simulink model "Pendulum_Model"  (R2015a)
settings: Solver=ode45  StartTime=0.0  StopTime=50  RelTol=1e-3
undefined symbols (not defined in the file or in its folder): F_fan, g, k, l, m
libraries: simulink_extras x1
settings Model: CovSFcnEnable=off  Creator=shivjr  LastModifiedBy=shivjr
settings DebuggingCC: SolverPrmCheckMsg=warning

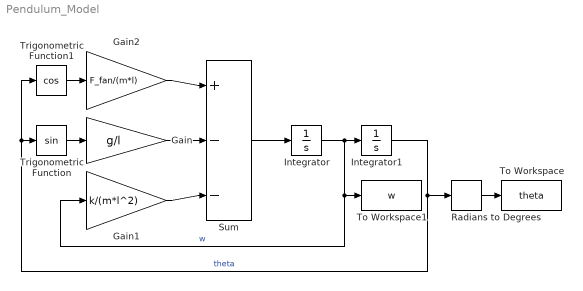
== system Pendulum_Model ==
  Gain : Gain  Gain=g/l
  Gain1 : Gain  Gain=k/(m*l^2)
  Gain2 : Gain  Gain=F_fan/(m*l)
  Integrator : Integrator
  Integrator1 : Integrator
  Radians to Degrees : simulink_extras/Transformations/Radians to Degrees
  Sum : Sum  Inputs=+|-|-
  To Workspace : ToWorkspace  VariableName=theta  SaveFormat=Timeseries  SampleTime=-1
  To Workspace1 : ToWorkspace  VariableName=w  SaveFormat=Timeseries  SampleTime=-1
  Trigonometric Function : Trigonometry
  Trigonometric Function1 : Trigonometry  Operator=cos
  wires:
  Trigonometric Function/1 -> Gain/1
  Trigonometric Function1/1 -> Gain2/1
  Gain2/1 -> Sum/1
  Gain/1 -> Sum/2
  Gain1/1 -> Sum/3
  Integrator1/1 -> Radians to Degrees/1, Trigonometric Function1/1, Trigonometric Function/1  "theta"
  Integrator/1 -> To Workspace1/1, Gain1/1, Integrator1/1  "w"
  Sum/1 -> Integrator/1
  Radians to Degrees/1 -> To Workspace/1
